simulink model "concatTest"  (R2015a)
settings: Solver=ode45  StartTime=0.0  StopTime=10.0  RelTol=1e-3
settings Model: Creator=shohei  LastModifiedBy=shohei

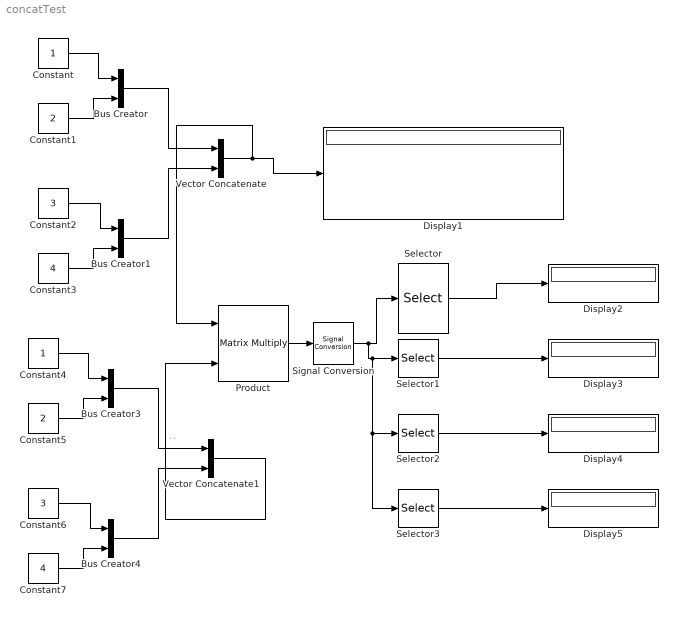
== system concatTest ==
  Bus Creator{,1,3..4} (4 alike) : BusCreator  Inputs=2
  Constant : Constant
  Constant1 : Constant  Value=2
  Constant2 : Constant  Value=3
  Constant3 : Constant  Value=4
  Constant4 : Constant
  Constant5 : Constant  Value=2
  Constant6 : Constant  Value=3
  Constant7 : Constant  Value=4
  Display{1..5} (5 alike) : Display
  Product : Product  Multiplication=Matrix(*)
  Selector : Selector  InputPortWidth=4
  Selector1 : Selector  InputPortWidth=4  Indices=2
  Selector2 : Selector  InputPortWidth=4  Indices=3
  Selector3 : Selector  InputPortWidth=4  Indices=4
  Signal Conversion : SignalConversion  ConversionOutput=Nonvirtual bus
  Vector Concatenate : Concatenate  Mode=Multidimensional array  ConcatenateDimension=2
  Vector Concatenate1 : Concatenate  Mode=Multidimensional array  ConcatenateDimension=2
  wires:
  Constant2/1 -> Bus Creator1/1
  Constant3/1 -> Bus Creator1/2
  Constant/1 -> Bus Creator/1
  Constant1/1 -> Bus Creator/2
  Bus Creator/1 -> Vector Concatenate/1
  Bus Creator1/1 -> Vector Concatenate/2
  Constant6/1 -> Bus Creator4/1
  Constant7/1 -> Bus Creator4/2
  Constant4/1 -> Bus Creator3/1
  Constant5/1 -> Bus Creator3/2
  Bus Creator3/1 -> Vector Concatenate1/1
  Bus Creator4/1 -> Vector Concatenate1/2
  Vector Concatenate/1 -> Product/1, Display1/1
  Vector Concatenate1/1 -> Product/2  "``"
  Selector/1 -> Display2/1
  Selector1/1 -> Display3/1
  Selector2/1 -> Display4/1
  Selector3/1 -> Display5/1
  Product/1 -> Signal Conversion/1
  Signal Conversion/1 -> Selector3/1, Selector2/1, Selector1/1, Selector/1
